simulink model "ex_blocchi_elementi_continui"  (R2024b)
settings: Solver=VariableStepAuto  StartTime=0.0  StopTime=10.0  RelTol=1e-3
libraries: simulink x1

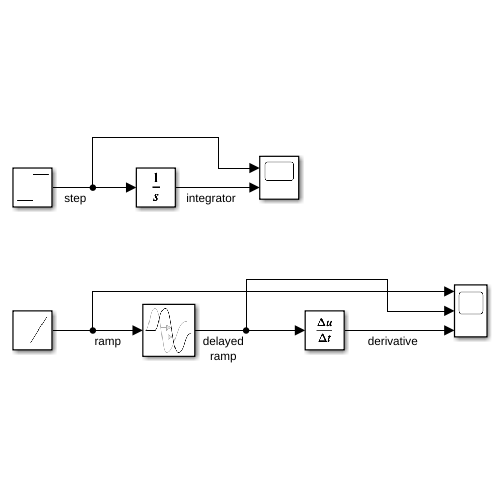
[thumbnail: Simulink's stored preview of the top-level diagram]
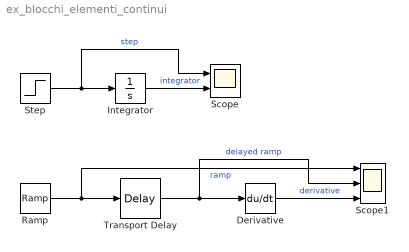
== system ex_blocchi_elementi_continui ==
  Derivative : Derivative
  Integrator : Integrator
  Ramp : simulink/Sources/Ramp  slope=1  start=0  InitialOutput=0
  Scope : Scope  NumInputPorts=2
  Scope1 : Scope  NumInputPorts=3
  Step : Step  SampleTime=0
  Transport Delay : TransportDelay
  wires:
  Step/1 -> Scope/1, Integrator/1  "step"
  Integrator/1 -> Scope/2  "integrator"
  Ramp/1 -> Scope1/1, Transport Delay/1  "ramp"
  Derivative/1 -> Scope1/3  "derivative"
  Transport Delay/1 -> Scope1/2, Derivative/1  "delayed ramp"
